simulink model "IZODROM"  (R2017a)
settings: Solver=VariableStepAuto  StartTime=0.0  StopTime=10.0  MaxStep=0.001000001  MinStep=0.001  RelTol=1e-5
undefined symbols (not defined in the file): k, T, w
settings Model: Creator=User  LastModifiedBy=User

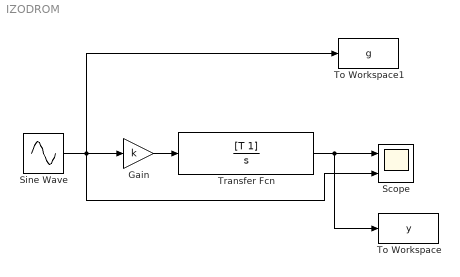
== system IZODROM ==
  Gain : Gain  Gain=k
  Scope : Scope  NumInputPorts=2
  Sine Wave : Sin  Frequency=w  SampleTime=0
  To Workspace : ToWorkspace  VariableName=y  SampleTime=-1
  To Workspace1 : ToWorkspace  VariableName=g  SampleTime=-1
  Transfer Fcn : TransferFcn  Numerator=[T 1]  Denominator=[1 0]
  wires:
  Transfer Fcn/1 -> To Workspace/1, Scope/1
  Sine Wave/1 -> Scope/2, To Workspace1/1, Gain/1
  Gain/1 -> Transfer Fcn/1
